simulink model "Copy_of_Single_track_Drift_model"  (R2024b)
settings: Solver=FixedStepAuto  StartTime=0.0  StopTime=10.0  RelTol=1e-3
model workspace (MAT data in the model file):
  x0 = [0; 0; 0; 1e-06; 0; 0; 0; 0; 0.0001]
values from neighbouring files (symbols this model uses):
  Q = diag([0.2, 0.2, 0.01, 0.5, 0.3, 0.0001, 0.001, 0, 0.05])    [Copy_of_bicycleModelParam.m]    (also in bicycleModelParam.m = [0.8 0.2; 0.4 0.8])
settings Model: Creator=fanny  LastModifiedBy=fanny
settings OptimizationCC: BlockReduction=off  DefaultParameterBehavior=Inlined  BufferReuse=off

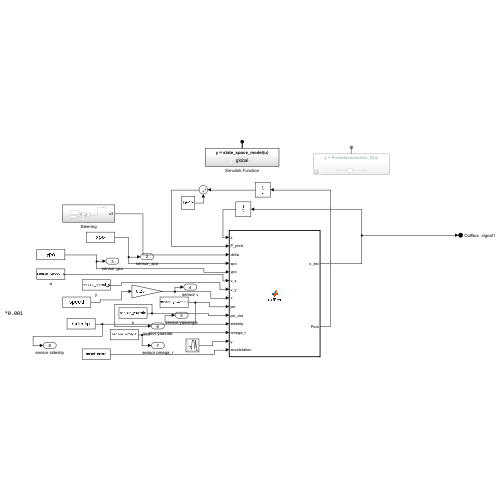
[thumbnail: Simulink's stored preview of the top-level diagram]
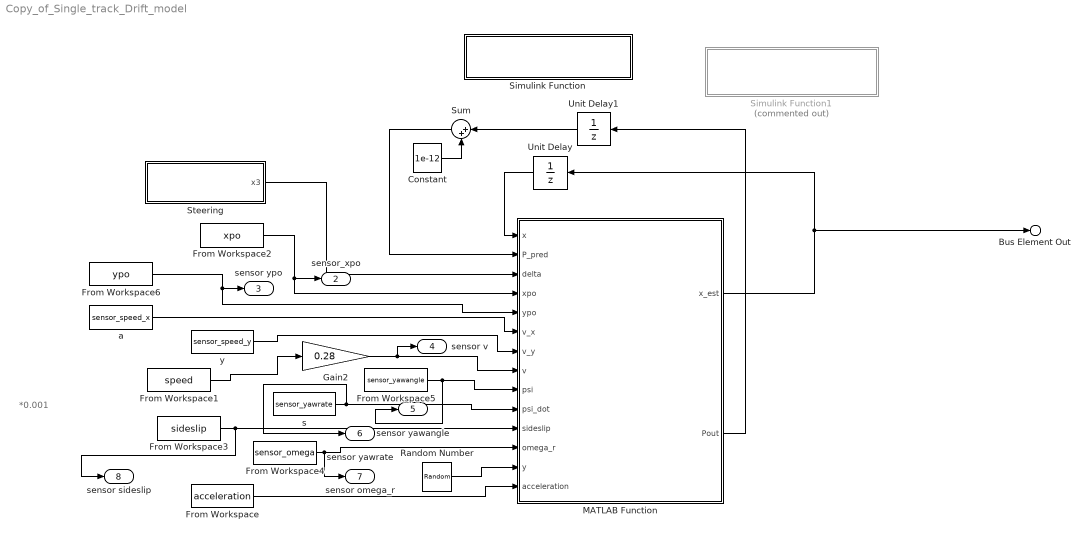
== system Copy_of_Single_track_Drift_model ==
  note: *0.001
  Constant : Constant  Value=1e-12
  From Workspace : FromWorkspace  VariableName=acceleration
  From Workspace1 : FromWorkspace  VariableName=speed  SampleTime=-1  OutputAfterFinalValue=Holding final value
  From Workspace2 : FromWorkspace  VariableName=xpo
  From Workspace3 : FromWorkspace  VariableName=sideslip  SampleTime=-1
  From Workspace4 : FromWorkspace  VariableName=sensor_omega  SampleTime=-1
  From Workspace5 : FromWorkspace  VariableName=sensor_yawangle  SampleTime=-1
  From Workspace6 : FromWorkspace  VariableName=ypo
  Gain2 : Gain  Gain=0.28
  MATLAB Function : MATLAB Function  TreatAsAtomicUnit=on  SystemSampleTime=0.001
  Random Number : RandomNumber  Variance=0.001  SampleTime=0.001
  Simulink Function : Subsystem  TreatAsAtomicUnit=on
  Simulink Function1 : Subsystem  Commented=on  TreatAsAtomicUnit=on
  Steering : Subsystem
  Sum : Sum  Inputs=|++
  Unit Delay : UnitDelay  InitialCondition=x0  SampleTime=-1  HasFrameUpgradeWarning=on
  Unit Delay1 : UnitDelay  InitialCondition=Q  SampleTime=-1  HasFrameUpgradeWarning=on
  a : FromWorkspace  VariableName=sensor_speed_x  SampleTime=-1
  s : FromWorkspace  VariableName=sensor_yawrate  SampleTime=-1
  y : FromWorkspace  VariableName=sensor_speed_y  SampleTime=-1
  Bus Element Out : Outport  PortName=OutBus  Element=signal1
  sensor_xpo : Outport  Port=2
  sensor ypo : Outport  Port=3
  sensor v : Outport  Port=4
  sensor yawangle : Outport  Port=5
  sensor yawrate : Outport  Port=6
  sensor omega_r : Outport  Port=7
  sensor sideslip : Outport  Port=8
  wires:
  MATLAB Function/1(x_est) -> Unit Delay/1, Bus Element Out/1
  Unit Delay/1 -> MATLAB Function/1(x)
  MATLAB Function/2(Pout) -> Unit Delay1/1
  Sum/1 -> MATLAB Function/2(P_pred)
  Constant/1 -> Sum/2
  From Workspace1/1 -> Gain2/1
  Unit Delay1/1 -> Sum/1
  From Workspace3/1 -> sensor sideslip/1, MATLAB Function/11(sideslip)
  s/1 -> sensor yawrate/1, MATLAB Function/10(psi_dot)
  a/1 -> MATLAB Function/6(v_x)
  y/1 -> MATLAB Function/7(v_y)
  Gain2/1 -> sensor v/1, MATLAB Function/8(v)
  From Workspace4/1 -> sensor omega_r/1, MATLAB Function/12(omega_r)
  From Workspace5/1 -> sensor yawangle/1, MATLAB Function/9(psi)
  Steering/1(x3) -> MATLAB Function/3(delta)
  Random Number/1 -> MATLAB Function/13(y)
  From Workspace/1 -> MATLAB Function/14(acceleration)
  From Workspace2/1 -> sensor_xpo/1, MATLAB Function/4(xpo)
  From Workspace6/1 -> MATLAB Function/5(ypo), sensor ypo/1

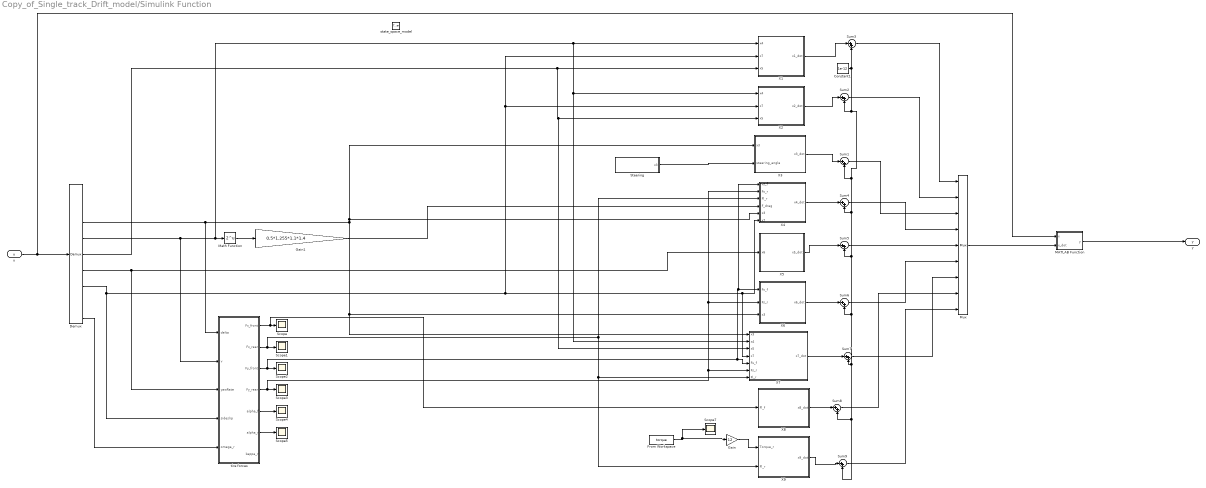
== system Copy_of_Single_track_Drift_model/Simulink Function ==
  state_space_model : TriggerPort  TriggerType=function-call  IsSimulinkFunction=on  FunctionName=state_space_model  VariantControl=(inherit)
  Constant1 : Constant  Value=1e-12
  Demux : Demux  Outputs=9
  From Workspace : FromWorkspace  VariableName=torque  SampleTime=-1  OutputAfterFinalValue=Holding final value
  Gain : Gain  Gain=12
  Gain1 : Gain  Gain=0.5*1.255*1.1*1.4
  MATLAB Function : MATLAB Function  TreatAsAtomicUnit=on
  Math Function : Math  Operator=2^u
  Mux : Mux  Inputs=9
  Scope{,1..5,7} (7 alike) : Scope
  Steering : Subsystem
  Sum{1..9} (9 alike) : Sum  Inputs=|++
  X1 : MATLAB Function  TreatAsAtomicUnit=on
  X2 : MATLAB Function  TreatAsAtomicUnit=on
  X3 : MATLAB Function  TreatAsAtomicUnit=on
  X4 : MATLAB Function  TreatAsAtomicUnit=on
  X5 : MATLAB Function  TreatAsAtomicUnit=on
  X6 : MATLAB Function  TreatAsAtomicUnit=on
  X7 : MATLAB Function  TreatAsAtomicUnit=on
  X8 : MATLAB Function  TreatAsAtomicUnit=on
  X9 : MATLAB Function  TreatAsAtomicUnit=on
  tire forces : MATLAB Function  TreatAsAtomicUnit=on
  u : ArgIn  DisableCoverage=on  PortDimensions=9  ArgumentName=u
  y : ArgOut  DisableCoverage=on  PortDimensions=9  ArgumentName=y
  wires:
  tire forces/5(alpha_f) -> Scope4/1
  tire forces/6(alpha_r) -> Scope5/1
  From Workspace/1 -> Scope7/1, Gain/1
  X8/1(x8_dot) -> Sum8/1
  X9/1(x9_dot) -> Sum9/1
  X7/1(x7_dot) -> Sum7/1
  Constant1/1 -> Sum3/2, Sum2/2, Sum1/2, Sum4/2, Sum5/2, Sum6/2, Sum8/2, Sum9/2, Sum7/2
  tire forces/3(Fy_front) -> X4/1(Fs_f), X6/1(Fs_f), X7/5(Fs_f), Scope2/1
  X2/1(x2_dot) -> Sum2/1
  X1/1(x1_dot) -> Sum3/1
  X3/1(x3_dot) -> Sum1/1
  X5/1(x5_dot) -> Sum5/1
  X6/1(x6_dot) -> Sum6/1
  tire forces/2(Fx_rear) -> X9/2(Fl_r), X7/7(Fl_r), X4/3(Fl_r), Scope1/1
  Math Function/1 -> Gain1/1
  tire forces/4(Fy_rear) -> X4/2(Fs_r), X6/2(Fs_r), X7/6(Fs_r), Scope3/1
  Gain/1 -> X9/1(Torque_r)
  X4/1(x4_dot) -> Sum4/1
  u/1 -> MATLAB Function/1(x), Demux/1
  Sum2/1 -> Mux/2
  Sum1/1 -> Mux/3
  Sum4/1 -> Mux/4
  Sum5/1 -> Mux/5
  Sum6/1 -> Mux/6
  Sum7/1 -> Mux/7
  Sum8/1 -> Mux/8
  Sum9/1 -> Mux/9
  Gain1/1 -> X4/4(F_drag)
  Demux/3 -> tire forces/1(delta), X4/5(x3), X3/1(x3), X7/1(x3), X6/3(x3)
  Demux/4 -> tire forces/2(v), Math Function/1, X1/1(x4), X2/1(x4), X7/2(x4)
  Demux/5 -> X7/3(x5), X2/3(x5), X1/3(x5)
  Demux/6 -> X5/1(x6), tire forces/3(yawRate)
  Demux/7 -> X2/2(x7), X1/2(x7), X4/6(x7), X7/4(x7), tire forces/4(sideslip)
  Demux/9 -> tire forces/5(omega_r)
  tire forces/1(Fx_front) -> X8/1(Fl_f), Scope/1
  Steering/1(x3) -> X3/2(steering_angle)
  Mux/1 -> MATLAB Function/2(x_dot)
  Sum3/1 -> Mux/1
  MATLAB Function/1(y) -> y/1

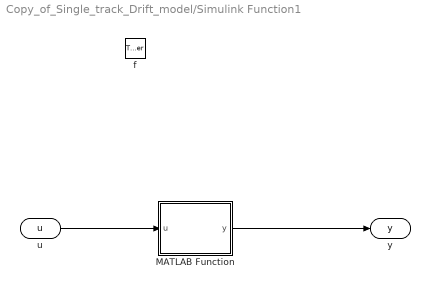
== system Copy_of_Single_track_Drift_model/Simulink Function1 ==
  f : TriggerPort  TriggerType=function-call  IsSimulinkFunction=on  FunctionName=Prozessrauschen_Q  FunctionVisibility=scoped  VariantControl=(inherit)
  MATLAB Function : MATLAB Function  TreatAsAtomicUnit=on
  u : ArgIn  DisableCoverage=on  ArgumentName=u
  y : ArgOut  DisableCoverage=on  PortDimensions=-1  ArgumentName=y
      settings: LockScale=on
  wires:
  u/1 -> MATLAB Function/1(u)
  MATLAB Function/1(y) -> y/1

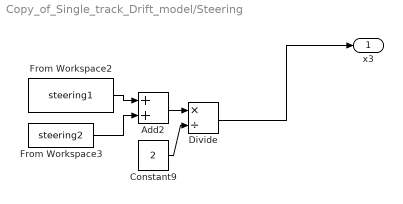
== system Copy_of_Single_track_Drift_model/Steering ==
  Add2 : Sum
  Constant9 : Constant  Value=2
  Divide : Product  Inputs=*/
  From Workspace2 : FromWorkspace  VariableName=steering1  SampleTime=-1
  From Workspace3 : FromWorkspace  VariableName=steering2  SampleTime=-1
  x3 : Outport
  wires:
  From Workspace3/1 -> Add2/2
  Constant9/1 -> Divide/2
  Divide/1 -> x3/1
  From Workspace2/1 -> Add2/1
  Add2/1 -> Divide/1

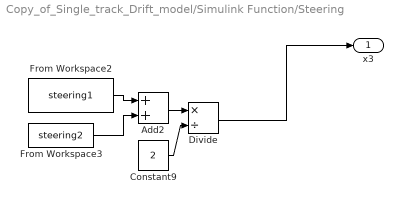
== system Copy_of_Single_track_Drift_model/Simulink Function/Steering ==
  Add2 : Sum
  Constant9 : Constant  Value=2
  Divide : Product  Inputs=*/
  From Workspace2 : FromWorkspace  VariableName=steering1  SampleTime=-1  OutputAfterFinalValue=Holding final value
  From Workspace3 : FromWorkspace  VariableName=steering2  SampleTime=-1  OutputAfterFinalValue=Holding final value
  x3 : Outport
  wires:
  From Workspace3/1 -> Add2/2
  Constant9/1 -> Divide/2
  Divide/1 -> x3/1
  From Workspace2/1 -> Add2/1
  Add2/1 -> Divide/1

== matlab function Copy_of_Single_track_Drift_model/Simulink Function/X8 ==
  data: x8_dot output; Fl_f input
function x8_dot = compute_omega_f_dot(Fl_f)
% Eingaben:
% Fl_f: Längskraft an der Vorderachse
% Iy_w: Trägheitsmoment des Rades
%
% Ausgabe:
% x8_dot: Ableitung von x8
Rw = 0.26;
Iw = 7*Rw^2;
% Zustandsgleichung für x8

x8_dot = 0;
end

== matlab function Copy_of_Single_track_Drift_model/Simulink Function/X9 ==
  data: x9_dot output; Torque_r input; Fl_r input
function x9_dot = compute_omega_r_dot(Torque_r, Fl_r)
% Eingaben:
% Torque_r: Antriebsmoment an der Hinterachse
% Fl_r: Längskraft an der Hinterachse
% Iy_w: Trägheitsmoment des Rades
%
% Ausgabe:
% x9_dot: Ableitung von x9
Rw = 0.26;
Iw = 10*Rw^2;

% Zustandsgleichung für x9
x9_dot = (1 / Iw) * ( -Torque_r + (Fl_r/2 * Rw));
end

== matlab function Copy_of_Single_track_Drift_model/Simulink Function/tire forces ==
  data: delta input; v input; Fx_front output; Fx_rear output; yawRate input; sideslip input; Fy_front output; Fy_rear output; omega_r input; alpha_f output; alpha_r output; kappa_r output
function [Fx_front, Fx_rear, Fy_front, Fy_rear, alpha_f, alpha_r, kappa_r] = calculateTireForces(delta, v, yawRate, sideslip, omega_r)
    % Berechnet die Reifenkräfte basierend auf Fahrzeugparametern und dynamischen Werten
    Fz = 2900 / 4;
    gamma = 0.0;
    Rw = 0.26035; % Reifenradius [m]
    vx = cos(delta)*v;
    L = 1.570; %[m] wheel base
    lf = 0.874; %[m] distance from center of mass to front axle
    lr = L-lf; %[m] distance from center of mass to rear axle

    % Longitudinal parameters
    pCx1 = 1.839;
    pDx1 = 1.1387;
    pKx1 = 18.886;
    pEx1 = 0.62727;
    pHx1 = -0.00033912;
    pVx1 = -4.638e-006;

    % Lateral parameters
    pCy1 = 1.322298;
    pDy1 = 1.216919;
    pKy1 = -19.79695;
    pEy1 = -0.637732;
    pHy1 = 0.00114529;
    pVy1 = 0.0375659;

    % Calculate slip angle alpha for both axles
    alpha_f = atan2(v * sin(sideslip) + yawRate * lf, v * cos(sideslip)) - delta;
    alpha_r = atan2(v * sin(sideslip) - yawRate * lr, v * cos(sideslip));
    alpha_r(isnan(alpha_r)) = 0;
    alpha_f(isnan(alpha_f)) = 0;
    % Calculate longitudinal slip kappa for both axles

    kappa_r = ((vx - Rw * omega_r) / vx); %original Pacejka 2002 paper
    % Calculate longitudinal forces (Fx)
    SHx = pHx1;
    SVx = Fz * pVx1;
    
    Fx_r = calculateFx(kappa_r, SHx, SVx, Fz, pDx1, pCx1, pEx1, pKx1);

    % Calculate lateral forces (Fy)
    SHy = pHy1 + gamma * 0.044112; % pHy3 from the VI-Grade tire file
    SVy = Fz * (pVy1 + gamma * -0.3293);

    Fy_f = calculateFy(alpha_f, SHy, SVy, Fz, pDy1, pCy1, pEy1, pKy1, gamma);
    Fy_r = calculateFy(alpha_r, SHy, SVy, Fz, pDy1, pCy1, pEy1, pKy1, gamma);

    % Combine forces for front and rear
    Fx_front = 0;
    Fx_rear = 2 * Fx_r;
    Fy_front = 2 * Fy_f - 21.6;
    Fy_rear = 2 * Fy_r - 21.6;

end

function Fx = calculateFx(kappa, SHx, SVx, Fz, pDx1, pCx1, pEx1, pKx1)
    kappa_x = kappa + SHx;
    mu_x = pDx1;
    Dx = mu_x * Fz;
    Cx = pCx1;
    Kx = Fz * pKx1;
    Bx = Kx / (Cx * Dx);
    Fx = Dx * sin(Cx * atan(Bx * kappa_x - pEx1 * (Bx * kappa_x - atan(Bx * kappa_x)))) + SVx;
end

function Fy = calculateFy(alpha, SHy, SVy, Fz, pDy1, pCy1, pEy1, pKy1, gamma)
    alpha_y = alpha + SHy;
    mu_y = pDy1 * (1 - (-2.8821) * gamma^2);
    Dy = mu_y * Fz;
    Cy = pCy1;
    Ky = Fz * pKy1;
    By = Ky / (Cy * Dy);
    Fy = Dy * sin(Cy * atan(By * alpha_y - pEy1 * (By * alpha_y - atan(By * alpha_y)))) + SVy;
end

== matlab function Copy_of_Single_track_Drift_model/MATLAB Function ==
  data: x input; P_pred input; delta input; xpo input; ypo input; v_x input; v_y input; v input; psi input; psi_dot input; sideslip input; omega_r input; x_est output; y input; Pout output; acceleration input
function [x_est, Pout] = ukfFcn(x, P_pred, delta,xpo, ypo, v_x, v_y, v,  psi, psi_dot, sideslip,  omega_r, y, acceleration)
    % Unscented Kalman Filter Implementation
    % x: Current state estimate [position; velocity]
    % P: Current state covariance matrix
    % u: Control input (acceleration)
    % y: Measurement (position)
    % Q: Process noise covariance matrix
    % R: Measurement noise covariance matrix
    % x_est: Updated state estimate
    % P: Updated state covariance matrix
    
    y = [xpo;
        ypo;
        delta;
        v;
        psi;
        psi_dot;
        sideslip;
        0;
        omega_r;];



    R = [0.0001;
        0.0001;
        0.001;
        0.0001;
        0.0001;
        0.00000001;
        0.000000001;
        0;
        0.000001;];
    

    % Unscented Transform Parameters
    n = numel(x); % Number of states
    alpha = 0.001; % Spread of sigma points
    kappa = 0;    % Secondary scaling parameter
    beta = 2;     % Optimal for Gaussian distributions
    lambda = alpha^2 * (n + kappa) - n; % Scaling parameter
    %gamma = sqrt(n + lambda); % Scaling factor
    %L = chol(P, 'lower'); 


    % Generate Sigma Points
    % Sigma points are selected around the current mean x
    sigmaPoints = zeros(n, 2*n+1);
    sigmaPoints(:,1) = x;
    P_pred(isnan(P_pred)) = 0;
    state_space_model(x);
    for i = 1:n
        sigmaPoints(:,2*i) = x + sqrt(abs((n + lambda) * P_pred(:, i)));
        sigmaPoints(:,2*i+1) = x - sqrt(abs((n + lambda) * P_pred(:, i)));
    end
    %disp(sigmaPoints(:,3:5));
    sigmaPoints(isnan(sigmaPoints)) = 0;
    % Predict Step
    % Propagate each sigma point through the state transition function
    sigmaPointsPredicted = zeros(size(sigmaPoints));

    for i = 1:2*n+1
        sigmaPointsPredicted(:, i) = state_space_model(sigmaPoints(:, i));
    end
    %disp(sigmaPointsPredicted(:,3:6));
    % Predicted Mean and Covariance
    weightsMean = zeros(1,2*n+1);
    %weightsMean(1,1) = lambda / (n+lambda); 
    weightsMean(1,2:2*n+1) = 1/18;
    weightsCov = weightsMean;


    x_pred = sigmaPointsPredicted * weightsMean';
    %disp(x_pred);
    for i = 1:2*n+1
        diff_pred = sigmaPointsPredicted(:, i) - x_pred;
        P_pred = P_pred + weightsCov(i) * (diff_pred * diff_pred');
    end

    % Measurement Update Step
    % Transform the predicted sigma points through the measurement function
    sigmaPointsMeasurements = sigmaPoints;
    %for i = 1:2*n+1
    %    sigmaPointsMeasurements(:, i) = measurementFcn(sigmaPoints(:, i), v_x, v_y, psi_dot, acceleration);
    %    sigmaPointsMeasurements(isnan(sigmaPointsMeasurements)) = 0;
    %end

    % Predicted Measurement Mean and Covariance
    Pyy = zeros(n, n);
    y_pred = sigmaPointsMeasurements * weightsMean'; % Predicted measurement mean
     % Initialize with measurement noise covariance
    for i = 1:2*n+1
        diff_meas = sigmaPointsMeasurements(:, i) - y_pred;
        Pyy = Pyy + weightsCov(i) * (diff_meas * diff_meas') + R;
    end

    % Cross-Covariance between State and Measurement
    Pxy = zeros(n, n);
    for i = 1:2*n+1
        stateDiff = sigmaPointsPredicted(:, i) - x_pred;
        measurementDiff = sigmaPointsMeasurements(:, i) - y_pred;
        Pxy = Pxy + weightsCov(i) * (stateDiff * measurementDiff');
    end

    % Kalman Gain
    Pyy(isnan(Pyy)) = 0;
    K = Pxy / Pyy;
    K(isnan(K)) = 0;
    % Update State and Covariance
    ys = y - y_pred;
    gain = K * ys;
    x_est = x_pred + gain; % Updated state estimate
    P_pred(isnan(P_pred)) = 0.0000001;
    Pout = P_pred - K * Pyy * K'; % Updated covariance matrix
end

function y = measurementFcn(x)
    % Measurement function
    % x: Current state
    % u: Measurement (position only in this example)
    
    % Assume we measure only position
    x(1) = x(1) + x(4)*sin(x(7)) * 0.001;
    x(2) = x(2) + x(4)*cos(x(7)) * 0.001;
    x(5) = x(5) + x(6)*0.001;
    x(7) = atan2(lh * tan(x(3)), L);
 
    x(isnan(x)) = 0;

    y = x;
end

== matlab function Copy_of_Single_track_Drift_model/Simulink Function/MATLAB Function ==
  data: x input; x_dot input; y output
function y = fcn(x, x_dot)


x2 = x + x_dot * 0.001; 
y = x2;

== matlab function Copy_of_Single_track_Drift_model/Simulink Function1/MATLAB Function ==
  data: u input; y output
function y  = fcn(u)
% Prozessrauschmatrix Q für das Single-Track-Drift-Modell
% Zustandsvektor: [sx, sy, delta, v, Psi, Psi_dot, beta, omega_f, omega_r]

% Definiere die Varianzen für unabhängiges Rauschen
sigma_sx = 0.1;       % Position x [m]
sigma_sy = 0.1;       % Position y [m]
sigma_delta = 0.001;  % Lenkwinkel [rad]
sigma_v = 0.5;        % Geschwindigkeit [m/s]
sigma_Psi = 0.01;     % Gierwinkel [rad]
sigma_Psi_dot = 0.001; % Giergeschwindigkeit [rad/s]
sigma_beta = 0.0025;  % Schräglaufwinkel [rad]
sigma_omega_f = 0; % Radgeschwindigkeit vorne [rad/s]
sigma_omega_r = 0.05; % Radgeschwindigkeit hinten [rad/s]

% Interne Abhängigkeiten (z.B. Geschwindigkeit beeinflusst Position, Gier beeinflusst Geschwindigkeit)
corr_v_Psi_dot = 0.05; % Korrelation zwischen Geschwindigkeit und Giergeschwindigkeit
corr_beta_Psi = 0.03;  % Korrelation zwischen Schräglaufwinkel und Gierwinkel

% Initialisiere die Matrix Q als Nullmatrix
Q = zeros(9, 9);

% Diagonalelemente: Varianzen der Zustände
Q(1, 1) = sigma_sx^2;
Q(2, 2) = sigma_sy^2;
Q(3, 3) = sigma_delta^2;
Q(4, 4) = sigma_v^2;
Q(5, 5) = sigma_Psi^2;
Q(6, 6) = sigma_Psi_dot^2;
Q(7, 7) = sigma_beta^2;
Q(8, 8) = sigma_omega_f^2;
Q(9, 9) = sigma_omega_r^2;

% Off-Diagonalelemente: Abhängigkeiten zwischen Zuständen
Q(4, 6) = corr_v_Psi_dot * sqrt(sigma_v^2 * sigma_Psi_dot^2);
Q(6, 4) = Q(4, 6); % Symmetrisch

Q(7, 5) = corr_beta_Psi * sqrt(sigma_beta^2 * sigma_Psi^2);
Q(5, 7) = Q(7, 5); % Symmetrisch

y = Q;

== matlab function Copy_of_Single_track_Drift_model/Simulink Function/X1 ==
  data: x4 input; x1_dot output; x7 input; x5 input
function x1_dot = compute_sx_dot(x4, x7, x5)
% Eingaben:
% x4, x7, x5: Zustände des Systems
%
% Ausgabe:
% x1_dot: Ableitung von x1

% Zustandsgleichung
x1_dot = 18/3.6 * cos(x7 + x5);
end

== matlab function Copy_of_Single_track_Drift_model/Simulink Function/X2 ==
  data: x4 input; x2_dot output; x7 input; x5 input
function x2_dot = compute_sy_dot(x4, x7, x5)
% Eingaben:
% x4: Zustand x4
% x7: Zustand x7
% x5: Zustand x5
%
% Ausgabe:
% x2_dot: Ableitung von x2

% Zustandsgleichung für x2
x2_dot = 18/3.6 * sin(x7 + x5);
end

== matlab function Copy_of_Single_track_Drift_model/Simulink Function/X3 ==
  data: x3 input; x3_dot output; steering_angle input
function x3_dot = compute_steering_angle_dot(x3, steering_angle)
% Eingaben:
% x3: Zustand x3
% u1: Eingangsgröße (z.B. Lenkwinkel)
%
% Ausgabe:
% x3_dot: Ableitung von x3

% Beispiel für f_steer: Die genaue Definition musst du anpassen
x3_dot = f_steer(x3, steering_angle);
end

function f = f_steer(x3, steering_angle)
% Hilfsfunktion für f_steer
% Definiere hier die Funktion f_steer abhängig von x3 und u1
f = steering_angle - x3; % Beispiel: Differenz zwischen Eingabe und Zustand
end

== matlab function Copy_of_Single_track_Drift_model/Simulink Function/X4 ==
  data: Fs_f input; Fs_r input; Fl_r input; F_drag input; x3 input; x4_dot output; x7 input
function x4_dot = compute_velocity_dot(Fs_f, Fs_r, Fl_r, F_drag, x3, x7)
% Eingaben:
% Fs_f: Seitliche Kraft vorne
% Fs_r: Seitliche Kraft hinten
% Fl_r: Längskraft hinten
% Fl_f: Längskraft vorne
% x3: Zustand steering angle
% x7: Zustand sideslip angle
%
% Ausgabe:
% x4_dot: Ableitung von velocity

m = 290; % in kg

% Zustandsgleichung für x4
v = (1/m) * (-Fs_f * sin(x3 - x7) + Fs_r * sin(x7) + Fl_r * cos(x7) - F_drag);

x4_dot = v;
end

== matlab function Copy_of_Single_track_Drift_model/Simulink Function/X5 ==
  data: x6 input; x5_dot output
function x5_dot = compute_yaw_angle_dot(x6)
% Eingabe:
% x6: Zustand x6
%
% Ausgabe:
% x5_dot: Ableitung von x5

% Zustandsgleichung für x5
x5_dot = x6;
end

== matlab function Copy_of_Single_track_Drift_model/Simulink Function/X6 ==
  data: Fs_f input; Fs_r input; x3 input; x6_dot output
function x6_dot = compute_yaw_rate_dot(Fs_f, Fs_r, x3)
% Eingaben:
% Fs_f: Seitliche Kraft vorne
% Fs_r: Seitliche Kraft hinten
% Fl_f: Längskraft vorne
% x3: Zustand steering angle
% x4: Zustand velocity
%
% Ausgabe:
% x6_dot: Ableitung von x6
Iz = 124.403600; %[kg*m^2] yaw polar inertia 
L = 1.570; %[m] wheel base
l_f =0.874; %[m] distance from center of mass to front axle
l_r = L-l_f; %[m] distance from center of mass to rear axle

% Zustandsgleichung für x6
x6_dot = (1 / Iz) * (Fs_f * cos(x3) * l_f - Fs_r * l_r);
end

== matlab function Copy_of_Single_track_Drift_model/Simulink Function/X7 ==
  data: x3 input; x4 input; x5 input; x7 input; Fs_f input; Fs_r input; Fl_r input; x7_dot output
function x7_dot = compute_sideslip_angle_dot(x3, x4, x5, x7, Fs_f, Fs_r, Fl_r)
% Eingaben:
% x5: yawrate
% x4: velocity
% Fs_f: Seitliche Kraft vorne
% Fs_r: Seitliche Kraft hinten
% Fl_r: Längskraft hinten
% Fl_f: Längskraft vorne
% x3: steering angle
% x7: sideslip
%
% Ausgabe:
% x7_dot: Ableitung von x7
m = 290;
% Zustandsgleichung für x7
forces = (Fs_f * cos(x3 - x7) + Fs_r * cos(x7) - Fl_r * sin(x7));
x7_dot = -x5 + (1 / (m * x4)) * forces;
end
